simulink model "controls"  (R2020a)
settings: Solver=ode3  StartTime=0.0  StopTime=10.0  FixedStep=1/par.freq  RelTol=1e-3
undefined symbols (not defined in the file): INDI, INDI_DRF, par
libraries: eeGeneralControl x7, simulink x4
settings Model: Creator=Matthias  LastModifiedBy=sihao
settings DataIOCC: SaveOutput=off  SaveTime=off  ReturnWorkspaceOutputs=off
settings DebuggingCC: ModelReferenceExtraNoncontSigs=warning  ArithmeticOperatorsInVariantConditions=warning
settings ModelReferenceCC: ModelReferenceNumInstancesAllowed=Single
settings SFSimCC: CustomCodeUndefinedFunction=UseInterfaceOnly
settings GRTTargetCC: CombineOutputUpdateFcns=off  MatFileLogging=off

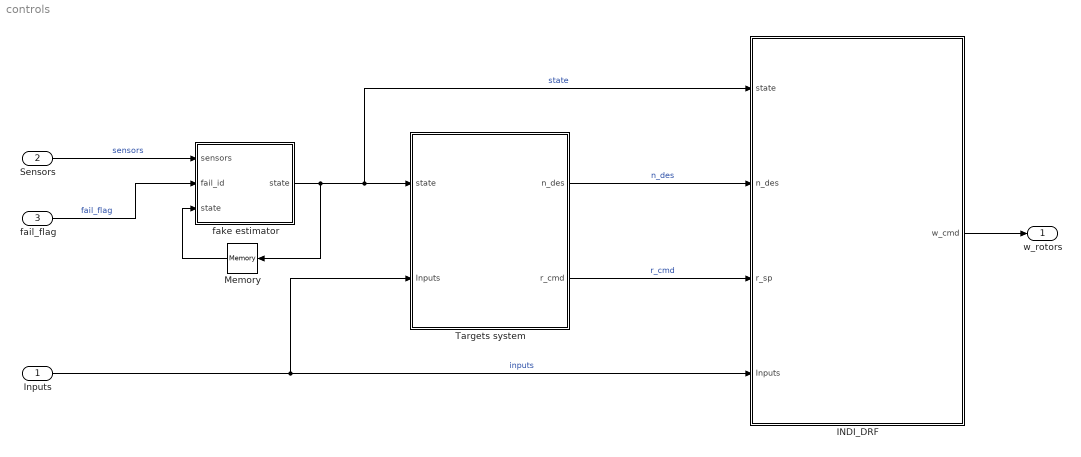
== system controls ==
  Inputs : Inport  OutDataTypeStr=Bus: inputsBus
  Sensors : Inport  Port=2  OutDataTypeStr=Bus: sensorsBus
  fail_flag : Inport  Port=3  OutDataTypeStr=double  PortDimensions=1
  INDI_DRF : Subsystem  AncestorBlock=INDI/INDI_DRF
  Memory : Memory
  Targets system : Subsystem
  "fake estimator " : MATLAB Function  TreatAsAtomicUnit=on
  w_rotors : Outport  VectorParamsAs1DForOutWhenUnconnected=off
  wires:
  fail_flag/1 -> "fake estimator "/2(fail_id)  "fail_flag"
  Targets system/2(r_cmd) -> INDI_DRF/3(r_sp)  "r_cmd"
  "fake estimator "/1(state) -> Memory/1, INDI_DRF/1(state), Targets system/1(state)  "state"
  Inputs/1 -> Targets system/2(Inputs), INDI_DRF/4(Inputs)  "inputs"
  INDI_DRF/1(w_cmd) -> w_rotors/1
  Targets system/1(n_des) -> INDI_DRF/2(n_des)  "n_des"
  Sensors/1 -> "fake estimator "/1(sensors)  "sensors"
  Memory/1 -> "fake estimator "/3("state ")

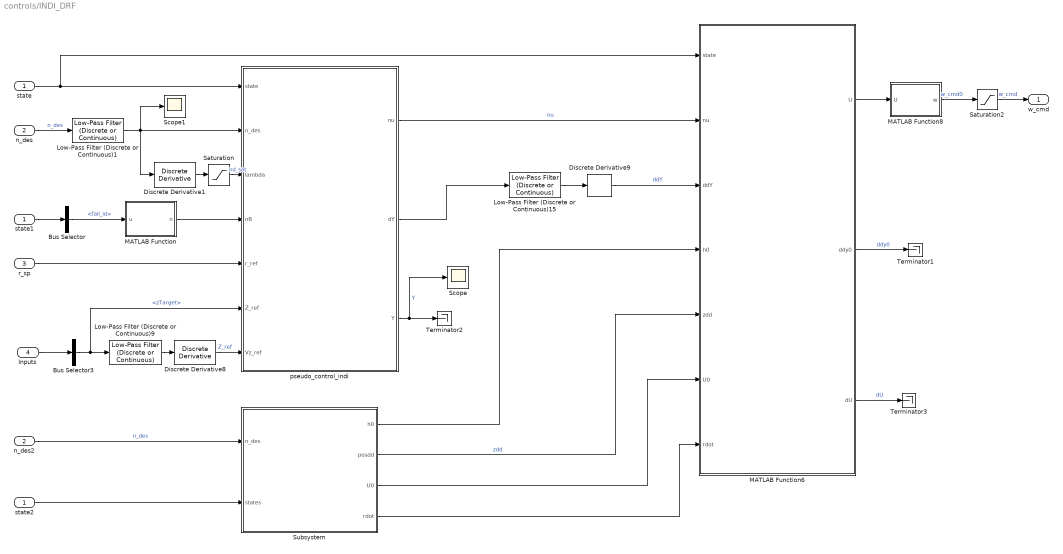
== system controls/INDI_DRF ==
  state : Inport
  n_des : Inport  Port=2  PortDimensions=3
  r_sp : Inport  Port=3
  Inputs : Inport  Port=4
  Bus Selector : BusSelector  OutputSignals=fail_id
  Bus Selector3 : BusSelector  OutputSignals=zTarget
  Discrete Derivative1 : simulink/Discrete/Discrete Derivative  gainval=1.0  ICPrevScaledInput=0.0  OutMin=[]  OutMax=[]  OutDataType=fixdt(1, 16)  OutScaling=2^-10  DoSatur=off
  Discrete Derivative8 : simulink/Discrete/Discrete Derivative  gainval=1.0  ICPrevScaledInput=0.0  OutMin=[]  OutMax=[]  OutDataType=fixdt(1, 16)  OutScaling=2^-10  DoSatur=off
  Discrete Derivative9 : simulink/Discrete/Discrete Derivative  gainval=1.0  ICPrevScaledInput=0.0  OutMin=[]  OutMax=[]  OutDataType=fixdt(1, 16)  OutScaling=2^-10  DoSatur=off
  Low-Pass Filter (Discrete or Continuous)1 : eeGeneralControl/Low-Pass Filter (Discrete or Continuous)  K=1  T=par.t_indi  B=inf  A=-inf  init_option=Inherited from block input  x0=0  Ts=-1
  Low-Pass Filter (Discrete or Continuous)15 : eeGeneralControl/Low-Pass Filter (Discrete or Continuous)  K=1  T=par.t_indi  B=inf  A=-inf  init_option=Inherited from block input  x0=0  Ts=-1
  Low-Pass Filter (Discrete or Continuous)9 : eeGeneralControl/Low-Pass Filter (Discrete or Continuous)  K=1  T=par.t_indi  B=inf  A=-inf  init_option=Inherited from block input  x0=0  Ts=-1
  MATLAB Function : MATLAB Function  TreatAsAtomicUnit=on
  MATLAB Function6 : MATLAB Function  TreatAsAtomicUnit=on
  MATLAB Function8 : MATLAB Function  TreatAsAtomicUnit=on
  Saturation : Saturate
  Saturation2 : Saturate  UpperLimit=par.w_max  LowerLimit=par.w_min
  Scope : Scope
  Scope1 : Scope
  Subsystem : Subsystem
  Terminator1 : Terminator
  Terminator2 : Terminator
  Terminator3 : Terminator
  n_des2 : InportShadow  Port=2  PortDimensions=3
  pseudo_control_indi : MATLAB Function  TreatAsAtomicUnit=on
  state1 : InportShadow
  state2 : InportShadow
  w_cmd : Outport  VectorParamsAs1DForOutWhenUnconnected=off
  wires:
  MATLAB Function6/1(U) -> MATLAB Function8/1(U)
  pseudo_control_indi/3(Y) -> Scope/1, Terminator2/1  "Y"
  Saturation/1 -> pseudo_control_indi/3(lambda)  "nd_sat"
  Discrete Derivative1/1 -> Saturation/1
  Low-Pass Filter (Discrete or Continuous)1/1 -> Scope1/1, Discrete Derivative1/1, pseudo_control_indi/2(n_des)
  MATLAB Function6/2(ddy0) -> Terminator1/1  "ddy0"
  state1/1 -> Bus Selector/1
  state/1 -> pseudo_control_indi/1(state), MATLAB Function6/1(state)
  state2/1 -> Subsystem/2(states)
  Bus Selector/1 -> MATLAB Function/1(u)  "<fail_id>"
  Subsystem/4(rdot) -> MATLAB Function6/7(rdot)
  Subsystem/3(U0) -> MATLAB Function6/6(U0)
  Subsystem/2(posdd) -> MATLAB Function6/5(zdd)  "zdd"
  Subsystem/1(h0) -> MATLAB Function6/4(h0)
  n_des2/1 -> Subsystem/1(n_des)  "n_des"
  Low-Pass Filter (Discrete or Continuous)15/1 -> Discrete Derivative9/1
  Discrete Derivative9/1 -> MATLAB Function6/3(ddY)  "ddY"
  pseudo_control_indi/2(dY) -> Low-Pass Filter (Discrete or Continuous)15/1
  Saturation2/1 -> w_cmd/1  "w_cmd"
  n_des/1 -> Low-Pass Filter (Discrete or Continuous)1/1  "n_des"
  MATLAB Function8/1(w) -> Saturation2/1  "w_cmd0"
  MATLAB Function/1(n) -> pseudo_control_indi/4(nB)
  pseudo_control_indi/1(nu) -> MATLAB Function6/2(nu)  "nu"
  Low-Pass Filter (Discrete or Continuous)9/1 -> Discrete Derivative8/1
  Bus Selector3/1 -> Low-Pass Filter (Discrete or Continuous)9/1, pseudo_control_indi/6(Z_ref)  "<zTarget>"
  Discrete Derivative8/1 -> pseudo_control_indi/7(Vz_ref)  "Z_ref"
  r_sp/1 -> pseudo_control_indi/5(r_ref)
  Inputs/1 -> Bus Selector3/1
  MATLAB Function6/3(dU) -> Terminator3/1  "dU"

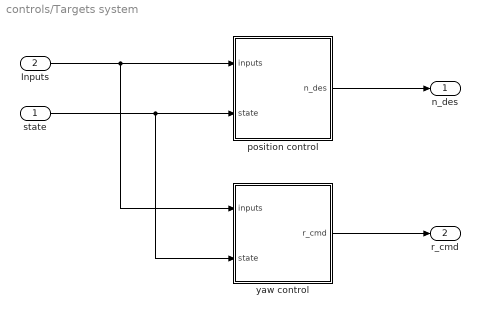
== system controls/Targets system ==
  state : Inport
  Inputs : Inport  Port=2
  position control : MATLAB Function  TreatAsAtomicUnit=on
  yaw control : MATLAB Function  TreatAsAtomicUnit=on
  n_des : Outport  VectorParamsAs1DForOutWhenUnconnected=off
  r_cmd : Outport  Port=2  VectorParamsAs1DForOutWhenUnconnected=off
  wires:
  yaw control/1(r_cmd) -> r_cmd/1
  Inputs/1 -> yaw control/1(inputs), position control/1(inputs)
  state/1 -> yaw control/2(state), position control/2(state)
  position control/1(n_des) -> n_des/1

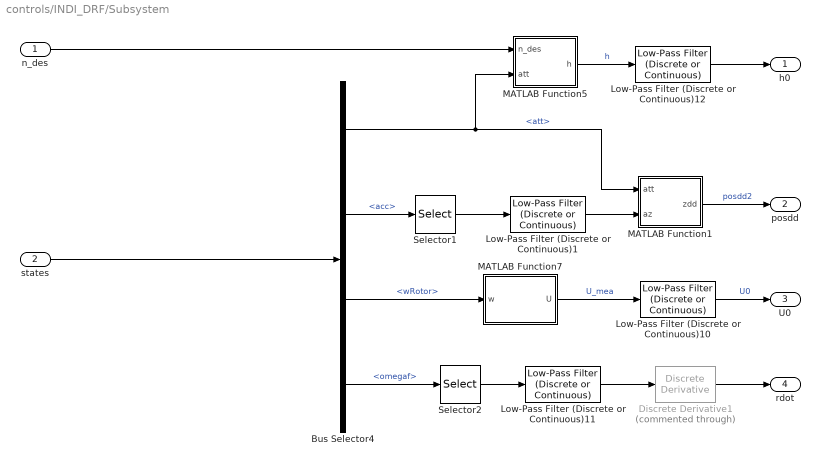
== system controls/INDI_DRF/Subsystem ==
  n_des : Inport
  states : Inport  Port=2
  Bus Selector4 : BusSelector  OutputSignals=att,acc,wRotor,omegaf
  Discrete Derivative1 : simulink/Discrete/Discrete Derivative  Commented=through  gainval=1.0  ICPrevScaledInput=0.0  OutMin=[]  OutMax=[]  OutDataType=fixdt(1, 16)  OutScaling=2^-10  DoSatur=off
  Low-Pass Filter (Discrete or Continuous){1,10..12} (4 alike) : eeGeneralControl/Low-Pass Filter (Discrete or Continuous)  K=1  T=par.t_indi  B=inf  A=-inf  init_option=Inherited from block input  x0=0  Ts=-1
  MATLAB Function1 : MATLAB Function  TreatAsAtomicUnit=on
  MATLAB Function5 : MATLAB Function  TreatAsAtomicUnit=on
  MATLAB Function7 : MATLAB Function  TreatAsAtomicUnit=on
  Selector1 : Selector  InputPortWidth=3  IndexOptions=Index vector (dialog)  Indices=3  OutputSizes=1
  Selector2 : Selector  InputPortWidth=3  IndexOptions=Index vector (dialog)  Indices=3  OutputSizes=1
  h0 : Outport  VectorParamsAs1DForOutWhenUnconnected=off
  posdd : Outport  Port=2  VectorParamsAs1DForOutWhenUnconnected=off
  U0 : Outport  Port=3  VectorParamsAs1DForOutWhenUnconnected=off
  rdot : Outport  Port=4  VectorParamsAs1DForOutWhenUnconnected=off
  wires:
  MATLAB Function1/1(zdd) -> posdd/1  "posdd2"
  Low-Pass Filter (Discrete or Continuous)1/1 -> MATLAB Function1/2(az)
  Selector1/1 -> Low-Pass Filter (Discrete or Continuous)1/1
  Bus Selector4/2 -> Selector1/1  "<acc>"
  n_des/1 -> MATLAB Function5/1(n_des)
  Low-Pass Filter (Discrete or Continuous)12/1 -> h0/1
  Low-Pass Filter (Discrete or Continuous)11/1 -> Discrete Derivative1/1
  Low-Pass Filter (Discrete or Continuous)10/1 -> U0/1  "U0"
  MATLAB Function7/1(U) -> Low-Pass Filter (Discrete or Continuous)10/1  "U_mea"
  Selector2/1 -> Low-Pass Filter (Discrete or Continuous)11/1
  MATLAB Function5/1(h) -> Low-Pass Filter (Discrete or Continuous)12/1  "h"
  states/1 -> Bus Selector4/1
  Bus Selector4/1 -> MATLAB Function1/1(att), MATLAB Function5/2(att)  "<att>"
  Bus Selector4/3 -> MATLAB Function7/1(w)  "<wRotor>"
  Bus Selector4/4 -> Selector2/1  "<omegaf>"
  Discrete Derivative1/1 -> rdot/1

== matlab function controls/INDI_DRF/pseudo_control_indi ==
  data: state input; n_des input; lambda input; nB input; r_ref input; Z_ref input; Vz_ref input; nu output; par parameter; dY output; Y output
function [nu,dY, Y] = pseudo_control_att_indi(state, n_des, lambda, nB, r_ref, Z_ref, Vz_ref, par)

[nu, dY, Y] = pseudo_control_att_indi(state, n_des, lambda, nB, r_ref, Z_ref, Vz_ref, par);

end

== matlab function controls/INDI_DRF/MATLAB Function ==
  data: u input; n output; par parameter
function n = fcn(u,par)

a = par.axis_tilt;

if par.DRF_enable == 0 || par.DRF_enable == 1 
    if u == 1
       n = [-a, a, -1];   
    elseif u == 2
       n = [-a, -a, -1];
    elseif u == 3
       n = [a, -a, -1];
    elseif u == 4
       n = [a, a, -1];
    else
       n = [0, 0, -1];    
    end
else
   n = [0, 0, -1];
end

== matlab function controls/Targets system/position control ==
  data: inputs input Bus: inputsBus; n_des output size=[1 3]; state input Bus: stateBus; par parameter
function n_des   = positionControl(inputs, state, par)

[n_des] = URpositionControl(inputs, state, par);

end

== matlab function controls/Targets system/yaw control ==
  data: inputs input Bus: inputsBus; r_cmd output; state input Bus: stateBus; par parameter
function r_cmd = yawControl(inputs, state, par)

[r_cmd] = URYawControl(inputs, state, par);

end

== matlab function controls/fake estimator  ==
  data: sensors input; fail_id input; state input Bus: stateBus; state output
function state  = fcn(sensors, fail_id, state)

state = UREstimators(sensors, fail_id, state);

end

== matlab function controls/INDI_DRF/MATLAB Function6 ==
  data: state input; nu input; ddY input; h0 input; zdd input; U0 input; rdot input; U output; par parameter; ddy0 output; dU output
function [U,ddy0,dU]  =  allocation_att_indi(state, nu, ddY, h0, zdd, U0, rdot, par)
    [U,ddy0,dU]  =  allocation_att_indi(state, nu, ddY, h0, zdd, U0, rdot, par);
end

== matlab function controls/INDI_DRF/Subsystem/MATLAB Function1 ==
  data: att input; az input; zdd output
function zdd = fcn(att,az)

phi = att(1);
theta = att(2);

zdd = az*cos(theta)*cos(phi) + 9.8124;

== matlab function controls/INDI_DRF/MATLAB Function8 ==
  data: U input; w output
function w = U2omega(U)
%#codegen

w = zeros(4,1);
w(1) = sqrt(abs(U(1)))*sign(U(1));
w(2) = sqrt(abs(U(2)))*sign(U(2));
w(3) = sqrt(abs(U(3)))*sign(U(3));
w(4) = sqrt(abs(U(4)))*sign(U(4));

end

== matlab function controls/INDI_DRF/Subsystem/MATLAB Function5 ==
  data: n_des input; att input; h output
function h = fcn(n_des, att)

phi = att(1);
theta = att(2);
psi = att(3);

R_IB = euler2Rot(phi,theta,psi);

h = R_IB \ n_des;

== matlab function controls/INDI_DRF/Subsystem/MATLAB Function7 ==
  data: w input; U output
function U = omega2U(w)
%#codegen

U = zeros(4,1);
U(1) = w(1)^2;
U(2) = w(2)^2;
U(3) = w(3)^2;
U(4) = w(4)^2;
end
